simulink model "sampleModel7293_pp_1_1"  (R2018a)
settings: Solver=VariableStepAuto  StartTime=0.0  StopTime=10.0  RelTol=1e-3
undefined symbols (not defined in the file): DiscIntNeverNeededParam
libraries: simulink x367
(part 2 of 12)

== system sampleModel7293_pp_1_1/cfblk166 ==
  cfblk1 : Inport
  Action Port : ActionPort  ActionType=then
  cfblk10 : UnitDelay  SampleTime=-1
  cfblk3 : DiscreteTransferFcn
  cfblk4 : DiscreteFir
  cfblk5 : Subsystem  TreatAsAtomicUnit=on
  cfblk6 : UnitDelay  SampleTime=-1
  cfblk7 : Subsystem  TreatAsAtomicUnit=on
  cfblk8 : simulink/Discrete/Transfer Fcn Real Zero  ZeroZ=0.75  ICPrevInput=0.0  DoSatur=off
      settings: SourceProductName=Simulink  SourceProductBaseCode=SL
  cfblk9 : DiscreteFilter
  cyemi_{96..103} (8 alike) : DataTypeConversion  OutDataTypeStr=double
  emi_1695 : Subsystem  TreatAsAtomicUnit=on
  emi_1697 : If  IfExpression=Inf <= u1
  emi_1698 : DataTypeConversion  OutDataTypeStr=double
  emi_1838 : Subsystem  TreatAsAtomicUnit=on
  emi_1840 : If  IfExpression=Inf <= u1
  emi_1841 : DataTypeConversion  OutDataTypeStr=double
  cfblk2 : Outport
  cfblk11 : Outport  Port=2
  cfblk12 : Outport  Port=3
  wires:
  cfblk4/1 -> cfblk12/1
  cyemi_96/1 -> cfblk10/1
  cfblk8/1 -> cyemi_96/1
  cyemi_97/1 -> cfblk3/1
  cfblk10/1 -> cyemi_97/1, emi_1698/1
  cyemi_98/1 -> cfblk4/1
  cfblk3/1 -> cyemi_98/1, emi_1841/1
  cfblk1/1 -> cyemi_99/1
  cyemi_100/1 -> cfblk6/1
  cfblk9/1 -> cyemi_100/1
  cyemi_102/1 -> cfblk8/1
  cfblk6/1 -> cyemi_102/1
  cyemi_103/1 -> cfblk9/1
  cyemi_99/1 -> cfblk5/1(emi_1693)
  cfblk5/1(emi_1694) -> cyemi_103/1, cyemi_101/1, cfblk2/1
  emi_1697/1 -> cfblk5/Action
  emi_1697/2 -> emi_1695/Action
  emi_1698/1 -> emi_1697/1
  cyemi_101/1 -> cfblk7/1(emi_1836)
  cfblk7/1(emi_1837) -> cfblk11/1
  emi_1840/1 -> cfblk7/Action
  emi_1840/2 -> emi_1838/Action
  emi_1841/1 -> emi_1840/1

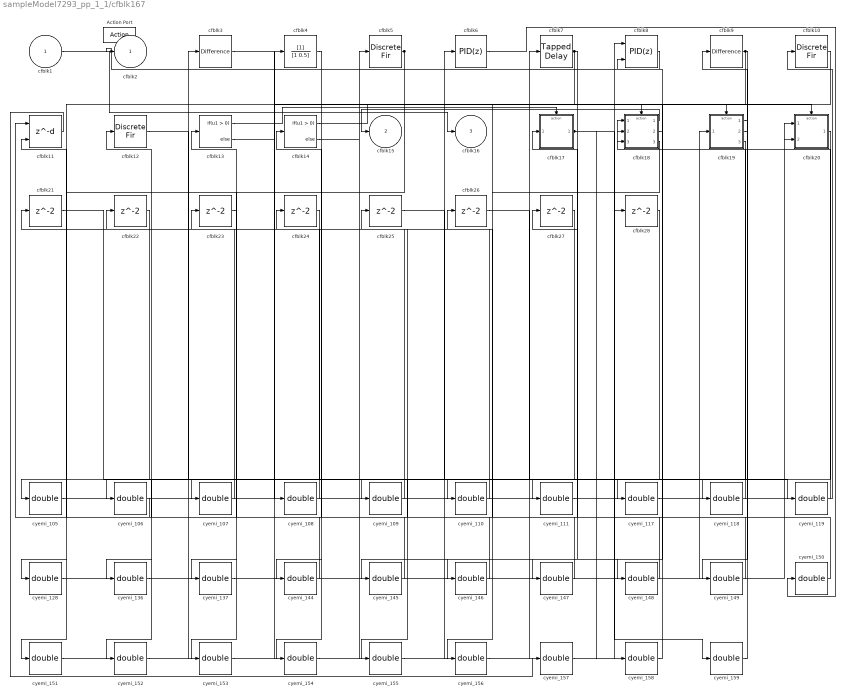
== system sampleModel7293_pp_1_1/cfblk167 ==
  cfblk1 : Inport
  Action Port : ActionPort  ActionType=else
  cfblk10 : DiscreteFir
  cfblk11 : Delay  DelayLengthSource=Input port
      settings: InputPortMap=u0,p1
  cfblk12 : DiscreteFir
  cfblk13 : If  SampleTime=1
  cfblk14 : If  SampleTime=1
  cfblk17 : Subsystem  TreatAsAtomicUnit=on
  cfblk18 : Subsystem  TreatAsAtomicUnit=on
  cfblk19 : Subsystem  TreatAsAtomicUnit=on
  cfblk20 : Subsystem  TreatAsAtomicUnit=on
  cfblk{21..28} (8 alike) : Delay
  cfblk3 : simulink/Discrete/Difference  ICPrevInput=0.0  OutMin=[]  OutMax=[]  OutDataTypeStr=double  OutputDataTypeScalingMode=double  OutDataType=fixdt(1, 16)  OutScaling=2^-10  DoSatur=off
  cfblk4 : DiscreteFilter
  cfblk5 : DiscreteFir
  cfblk6 : simulink/Continuous/PID Controller  Controller=PID  TimeDomain=Discrete-time  SampleTime=-1  IntegratorMethod=Forward Euler  FilterMethod=Forward Euler  Form=Parallel  UseFilter=on  ControllerParametersSource=internal  P=1  I=1  D=0  N=100  InitialConditionSource=internal  InitialConditionForIntegrator=0  InitialConditionForFilter=0  ExternalReset=none  LimitOutput=off  UpperSaturationLimit=inf  LowerSaturationLimit=-inf  LinearizeAsGain=off  AntiWindupMode=none  Kb=1  TrackingMode=off  Kt=1  PParamMin=[]  PParamMax=[]  IParamMin=[]  IParamMax=[]  DParamMin=[]  DParamMax=[]  NParamMin=[]  NParamMax=[]  KbParamMin=[]  KbParamMax=[]  KtParamMin=[]  KtParamMax=[]  POutMin=[]  POutMax=[]  IOutMin=[]  IOutMax=[]  DOutMin=[]  DOutMax=[]  NOutMin=[]  NOutMax=[]  KbOutMin=[]  KbOutMax=[]  KtOutMin=[]  KtOutMax=[]  IntegratorOutMin=[]  IntegratorOutMax=[]  FilterOutMin=[]  FilterOutMax=[]  SumOutMin=[]  SumOutMax=[]  SumI1OutMin=[]  SumI1OutMax=[]  SumI2OutMin=[]  SumI2OutMax=[]  SumI3OutMin=[]  SumI3OutMax=[]  SumDOutMin=[]  SumDOutMax=[]  SaturationOutMin=[]  SaturationOutMax=[]  IntegratorContinuousStateAttributes=''  IntegratorStateMustResolveToSignalObject=off  IntegratorRTWStateStorageClass=Auto  FilterContinuousStateAttributes=''  FilterStateMustResolveToSignalObject=off  FilterRTWStateStorageClass=Auto  DifferentiatorICPrevScaledInput=0  DifferentiatorOutMin=[]  DifferentiatorOutMax=[]  FilterDiffOutCoefMin=[]  FilterDiffOutCoefMax=[]  SumDenOutMin=[]  SumDenOutMax=[]  SumNumOutMin=[]  SumNumOutMax=[]  ReciprocalOutMin=[]  ReciprocalOutMax=[]  DivideOutMin=[]  DivideOutMax=[]  TunerSelectOption=Transfer Function Based (PID Tuner App)
  cfblk7 : simulink/Discrete/Tapped Delay  vinit=0.0  samptime=-1  NumDelays=1  DelayOrder=Oldest  includeCurrent=off
  cfblk8 : simulink/Continuous/PID Controller (2DOF)  Controller=PID  TimeDomain=Discrete-time  SampleTime=-1  IntegratorMethod=Forward Euler  FilterMethod=Forward Euler  Form=Parallel  UseFilter=on  ControllerParametersSource=internal  P=1  I=1  D=0  N=100  b=1  c=1  InitialConditionSource=internal  InitialConditionForIntegrator=0  InitialConditionForFilter=0  ExternalReset=none  LimitOutput=off  UpperSaturationLimit=inf  LowerSaturationLimit=-inf  LinearizeAsGain=off  AntiWindupMode=none  Kb=1  TrackingMode=off  Kt=1  PParamMin=[]  PParamMax=[]  IParamMin=[]  IParamMax=[]  DParamMin=[]  DParamMax=[]  NParamMin=[]  NParamMax=[]  bParamMin=[]  bParamMax=[]  cParamMin=[]  cParamMax=[]  KbParamMin=[]  KbParamMax=[]  KtParamMin=[]  KtParamMax=[]  POutMin=[]  POutMax=[]  IOutMin=[]  IOutMax=[]  DOutMin=[]  DOutMax=[]  NOutMin=[]  NOutMax=[]  bOutMin=[]  bOutMax=[]  cOutMin=[]  cOutMax=[]  KbOutMin=[]  KbOutMax=[]  KtOutMin=[]  KtOutMax=[]  IntegratorOutMin=[]  IntegratorOutMax=[]  FilterOutMin=[]  FilterOutMax=[]  SumOutMin=[]  SumOutMax=[]  Sum1OutMin=[]  Sum1OutMax=[]  Sum2OutMin=[]  Sum2OutMax=[]  Sum3OutMin=[]  Sum3OutMax=[]  SumI1OutMin=[]  SumI1OutMax=[]  SumI2OutMin=[]  SumI2OutMax=[]  SumI3OutMin=[]  SumI3OutMax=[]  SumDOutMin=[]  SumDOutMax=[]  SaturationOutMin=[]  SaturationOutMax=[]  IntegratorContinuousStateAttributes=''  IntegratorStateMustResolveToSignalObject=off  IntegratorRTWStateStorageClass=Auto  FilterContinuousStateAttributes=''  FilterStateMustResolveToSignalObject=off  FilterRTWStateStorageClass=Auto  DifferentiatorICPrevScaledInput=0  DifferentiatorOutMin=[]  DifferentiatorOutMax=[]  FilterDiffOutCoefMin=[]  FilterDiffOutCoefMax=[]  SumDenOutMin=[]  SumDenOutMax=[]  SumNumOutMin=[]  SumNumOutMax=[]  ReciprocalOutMin=[]  ReciprocalOutMax=[]  DivideOutMin=[]  DivideOutMax=[]  TunerSelectOption=Transfer Function Based (PID Tuner App)
  cfblk9 : simulink/Discrete/Difference  ICPrevInput=0.0  OutMin=[]  OutMax=[]  OutDataTypeStr=double  OutputDataTypeScalingMode=double  OutDataType=fixdt(1, 16)  OutScaling=2^-10  DoSatur=off
  cyemi_{105..111,117..119,128,136..137,144..159} (29 alike) : DataTypeConversion  OutDataTypeStr=double
  cfblk2 : Outport
  cfblk15 : Outport  Port=2
  cfblk16 : Outport  Port=3
  wires:
  cfblk1/1 -> cfblk16/1
  cfblk8/1 -> cfblk2/1
  cfblk17/1(cfblk2) -> cyemi_158/1, cyemi_159/1
  cfblk7/1 -> cyemi_111/1, cyemi_151/1
  cfblk18/1(cfblk2) -> cfblk15/1
  cfblk5/1 -> cyemi_105/1, cyemi_107/1
  cfblk9/1 -> cyemi_144/1, cyemi_148/1, cyemi_149/1
  cfblk13/1 -> cfblk17/Action
  cfblk13/2 -> cfblk18/Action
  cfblk14/1 -> cfblk19/Action
  cfblk14/2 -> cfblk20/Action
  cyemi_105/1 -> cfblk10/1
  cyemi_106/1 -> cfblk11/1
  cfblk19/1(cfblk2) -> cyemi_106/1
  cyemi_107/1 -> cfblk11/2
  cyemi_108/1 -> cfblk12/1
  cfblk3/1 -> cyemi_108/1
  cyemi_109/1 -> cfblk13/1
  cfblk19/2(cfblk8) -> cyemi_109/1
  cyemi_110/1 -> cfblk14/1
  cfblk12/1 -> cyemi_110/1
  cyemi_111/1 -> cfblk17/1(cfblk1)
  cyemi_117/1 -> cfblk18/1(cfblk1)
  cfblk21/1 -> cyemi_117/1
  cyemi_118/1 -> cfblk18/2(cfblk10)
  cfblk25/1 -> cyemi_118/1
  cyemi_119/1 -> cfblk18/3(cfblk11)
  cfblk26/1 -> cyemi_119/1
  cyemi_128/1 -> cfblk19/1(cfblk1)
  cfblk22/1 -> cyemi_128/1
  cyemi_136/1 -> cfblk20/1(cfblk1)
  cfblk27/1 -> cyemi_136/1
  cyemi_137/1 -> cfblk20/2(cfblk7)
  cfblk23/1 -> cyemi_137/1
  cyemi_144/1 -> cfblk21/1
  cyemi_145/1 -> cfblk22/1
  cfblk18/2(cfblk12) -> cyemi_145/1
  cyemi_146/1 -> cfblk23/1
  cfblk18/3(cfblk13) -> cyemi_146/1
  cyemi_147/1 -> cfblk24/1
  cfblk20/1(cfblk2) -> cyemi_147/1
  cyemi_148/1 -> cfblk25/1
  cyemi_149/1 -> cfblk26/1
  cyemi_150/1 -> cfblk27/1
  cfblk6/1 -> cyemi_150/1
  cyemi_151/1 -> cfblk28/1
  cyemi_152/1 -> cfblk3/1
  cfblk24/1 -> cyemi_152/1
  cyemi_153/1 -> cfblk4/1
  cfblk28/1 -> cyemi_153/1
  cyemi_154/1 -> cfblk5/1
  cfblk4/1 -> cyemi_154/1
  cyemi_155/1 -> cfblk6/1
  cfblk19/3(cfblk9) -> cyemi_155/1
  cyemi_156/1 -> cfblk7/1
  cfblk10/1 -> cyemi_156/1
  cyemi_157/1 -> cfblk8/1
  cfblk11/1 -> cyemi_157/1
  cyemi_158/1 -> cfblk8/2
  cyemi_159/1 -> cfblk9/1

== system sampleModel7293_pp_1_1/cfblk168 ==
  cfblk1 : Inport
  Action Port : ActionPort  ActionType=then
  cfblk3 : DiscreteStateSpace  SampleTime=-1
  cfblk4 : simulink/Continuous/PID Controller  Controller=PID  TimeDomain=Discrete-time  SampleTime=-1  IntegratorMethod=Forward Euler  FilterMethod=Forward Euler  Form=Parallel  UseFilter=on  ControllerParametersSource=internal  P=1  I=1  D=0  N=100  InitialConditionSource=internal  InitialConditionForIntegrator=0  InitialConditionForFilter=0  ExternalReset=none  LimitOutput=off  UpperSaturationLimit=inf  LowerSaturationLimit=-inf  LinearizeAsGain=off  AntiWindupMode=none  Kb=1  TrackingMode=off  Kt=1  PParamMin=[]  PParamMax=[]  IParamMin=[]  IParamMax=[]  DParamMin=[]  DParamMax=[]  NParamMin=[]  NParamMax=[]  KbParamMin=[]  KbParamMax=[]  KtParamMin=[]  KtParamMax=[]  POutMin=[]  POutMax=[]  IOutMin=[]  IOutMax=[]  DOutMin=[]  DOutMax=[]  NOutMin=[]  NOutMax=[]  KbOutMin=[]  KbOutMax=[]  KtOutMin=[]  KtOutMax=[]  IntegratorOutMin=[]  IntegratorOutMax=[]  FilterOutMin=[]  FilterOutMax=[]  SumOutMin=[]  SumOutMax=[]  SumI1OutMin=[]  SumI1OutMax=[]  SumI2OutMin=[]  SumI2OutMax=[]  SumI3OutMin=[]  SumI3OutMax=[]  SumDOutMin=[]  SumDOutMax=[]  SaturationOutMin=[]  SaturationOutMax=[]  IntegratorContinuousStateAttributes=''  IntegratorStateMustResolveToSignalObject=off  IntegratorRTWStateStorageClass=Auto  FilterContinuousStateAttributes=''  FilterStateMustResolveToSignalObject=off  FilterRTWStateStorageClass=Auto  DifferentiatorICPrevScaledInput=0  DifferentiatorOutMin=[]  DifferentiatorOutMax=[]  FilterDiffOutCoefMin=[]  FilterDiffOutCoefMax=[]  SumDenOutMin=[]  SumDenOutMax=[]  SumNumOutMin=[]  SumNumOutMax=[]  ReciprocalOutMin=[]  ReciprocalOutMax=[]  DivideOutMin=[]  DivideOutMax=[]  TunerSelectOption=Transfer Function Based (PID Tuner App)
  cfblk5 : DiscreteStateSpace  SampleTime=-1
  cfblk6 : DiscreteFir
  cfblk7 : Subsystem  TreatAsAtomicUnit=on
  cfblk9 : Delay
  cyemi_{161..167} (7 alike) : DataTypeConversion  OutDataTypeStr=double
  emi_1145 : Subsystem  TreatAsAtomicUnit=on
  emi_1147 : If  IfExpression=Inf <= u1
  emi_1148 : DataTypeConversion  OutDataTypeStr=double
  cfblk2 : Outport
  cfblk8 : Outport  Port=2
  wires:
  cfblk4/1 -> cfblk8/1
  cfblk6/1 -> cfblk2/1, cyemi_165/1, cyemi_166/1
  cyemi_161/1 -> cfblk3/1
  cfblk9/1 -> cyemi_161/1
  cyemi_162/1 -> cfblk4/1
  cfblk5/1 -> cyemi_162/1
  cyemi_163/1 -> cfblk5/1
  cfblk1/1 -> cyemi_163/1
  cyemi_164/1 -> cfblk6/1
  cfblk3/1 -> cyemi_164/1, emi_1148/1
  cyemi_167/1 -> cfblk9/1
  cyemi_165/1 -> cfblk7/1(emi_1142)
  cyemi_166/1 -> cfblk7/2(emi_1143)
  cfblk7/1(emi_1144) -> cyemi_167/1
  emi_1147/1 -> cfblk7/Action
  emi_1147/2 -> emi_1145/Action
  emi_1148/1 -> emi_1147/1

== system sampleModel7293_pp_1_1/cfblk169 ==
  cfblk1 : Inport
  cfblk12 : Inport  Port=2
  Action Port : ActionPort  ActionType=else
  cfblk10 : Delay
  cfblk11 : DiscreteFir
  cfblk3 : Subsystem  TreatAsAtomicUnit=on
  cfblk4 : simulink/Continuous/PID Controller  Controller=PID  TimeDomain=Discrete-time  SampleTime=-1  IntegratorMethod=Forward Euler  FilterMethod=Forward Euler  Form=Parallel  UseFilter=on  ControllerParametersSource=internal  P=1  I=1  D=0  N=100  InitialConditionSource=internal  InitialConditionForIntegrator=0  InitialConditionForFilter=0  ExternalReset=none  LimitOutput=off  UpperSaturationLimit=inf  LowerSaturationLimit=-inf  LinearizeAsGain=off  AntiWindupMode=none  Kb=1  TrackingMode=off  Kt=1  PParamMin=[]  PParamMax=[]  IParamMin=[]  IParamMax=[]  DParamMin=[]  DParamMax=[]  NParamMin=[]  NParamMax=[]  KbParamMin=[]  KbParamMax=[]  KtParamMin=[]  KtParamMax=[]  POutMin=[]  POutMax=[]  IOutMin=[]  IOutMax=[]  DOutMin=[]  DOutMax=[]  NOutMin=[]  NOutMax=[]  KbOutMin=[]  KbOutMax=[]  KtOutMin=[]  KtOutMax=[]  IntegratorOutMin=[]  IntegratorOutMax=[]  FilterOutMin=[]  FilterOutMax=[]  SumOutMin=[]  SumOutMax=[]  SumI1OutMin=[]  SumI1OutMax=[]  SumI2OutMin=[]  SumI2OutMax=[]  SumI3OutMin=[]  SumI3OutMax=[]  SumDOutMin=[]  SumDOutMax=[]  SaturationOutMin=[]  SaturationOutMax=[]  IntegratorContinuousStateAttributes=''  IntegratorStateMustResolveToSignalObject=off  IntegratorRTWStateStorageClass=Auto  FilterContinuousStateAttributes=''  FilterStateMustResolveToSignalObject=off  FilterRTWStateStorageClass=Auto  DifferentiatorICPrevScaledInput=0  DifferentiatorOutMin=[]  DifferentiatorOutMax=[]  FilterDiffOutCoefMin=[]  FilterDiffOutCoefMax=[]  SumDenOutMin=[]  SumDenOutMax=[]  SumNumOutMin=[]  SumNumOutMax=[]  ReciprocalOutMin=[]  ReciprocalOutMax=[]  DivideOutMin=[]  DivideOutMax=[]  TunerSelectOption=Transfer Function Based (PID Tuner App)
  cfblk5 : Subsystem  TreatAsAtomicUnit=on
  cfblk6 : Delay  DelayLengthSource=Input port
      settings: InputPortMap=u0,p1
  cfblk7 : Subsystem  TreatAsAtomicUnit=on
  cfblk8 : Subsystem  TreatAsAtomicUnit=on
  cfblk9 : Subsystem  TreatAsAtomicUnit=on
  cyemi_{170..180} (11 alike) : DataTypeConversion  OutDataTypeStr=double
  emi_1130 : Subsystem  TreatAsAtomicUnit=on
  emi_1132 : If  IfExpression=0 <= u1
  emi_{299,493,830,1133,1981} (5 alike) : DataTypeConversion  OutDataTypeStr=double
  emi_1978 : Subsystem  TreatAsAtomicUnit=on
  emi_1980 : If  IfExpression=0 <= u1
  emi_296 : Subsystem  TreatAsAtomicUnit=on
  emi_298 : If  IfExpression=-4.554546e-01 <= u1
  emi_490 : Subsystem  TreatAsAtomicUnit=on
  emi_492 : If  IfExpression=-4.554546e-01 <= u1
  emi_827 : Subsystem  TreatAsAtomicUnit=on
  emi_829 : If  IfExpression=0 <= u1
  cfblk2 : Outport
  cfblk13 : Outport  Port=2
  cfblk14 : Outport  Port=3
  wires:
  cfblk12/1 -> cyemi_171/1, cyemi_179/1, cyemi_180/1
  cfblk6/1 -> cfblk14/1, emi_1981/1
  cyemi_170/1 -> cfblk10/1
  cfblk1/1 -> cyemi_170/1
  cyemi_171/1 -> cfblk11/1
  cfblk4/1 -> cyemi_172/1
  cyemi_173/1 -> cfblk4/1
  cyemi_175/1 -> cfblk6/1
  cyemi_176/1 -> cfblk6/2
  cfblk10/1 -> cyemi_176/1
  cfblk11/1 -> cyemi_178/1, emi_299/1, emi_493/1
  cyemi_180/1 -> cfblk9/1(emi_294)
  cfblk9/1(emi_295) -> cyemi_177/1, cyemi_173/1
  emi_298/1 -> cfblk9/Action
  emi_298/2 -> emi_296/Action
  emi_299/1 -> emi_298/1
  cyemi_178/1 -> cfblk8/1(emi_487)
  cyemi_179/1 -> cfblk8/2(emi_488)
  cfblk8/1(emi_489) -> cyemi_174/1
  emi_492/1 -> cfblk8/Action
  emi_492/2 -> emi_490/Action
  emi_493/1 -> emi_492/1
  cyemi_174/1 -> cfblk5/1(emi_825)
  cfblk5/1(emi_826) -> cfblk2/1
  emi_829/1 -> cfblk5/Action
  emi_829/2 -> emi_827/Action
  emi_830/1 -> emi_829/1
  cyemi_172/1 -> cfblk3/1(emi_1128)
  cfblk3/1(emi_1129) -> cfblk13/1
  emi_1132/1 -> cfblk3/Action
  emi_1132/2 -> emi_1130/Action
  emi_1133/1 -> emi_1132/1
  cyemi_177/1 -> cfblk7/1(emi_1976)
  cfblk7/1(emi_1977) -> emi_1133/1, emi_830/1, cyemi_175/1
  emi_1980/1 -> cfblk7/Action
  emi_1980/2 -> emi_1978/Action
  emi_1981/1 -> emi_1980/1

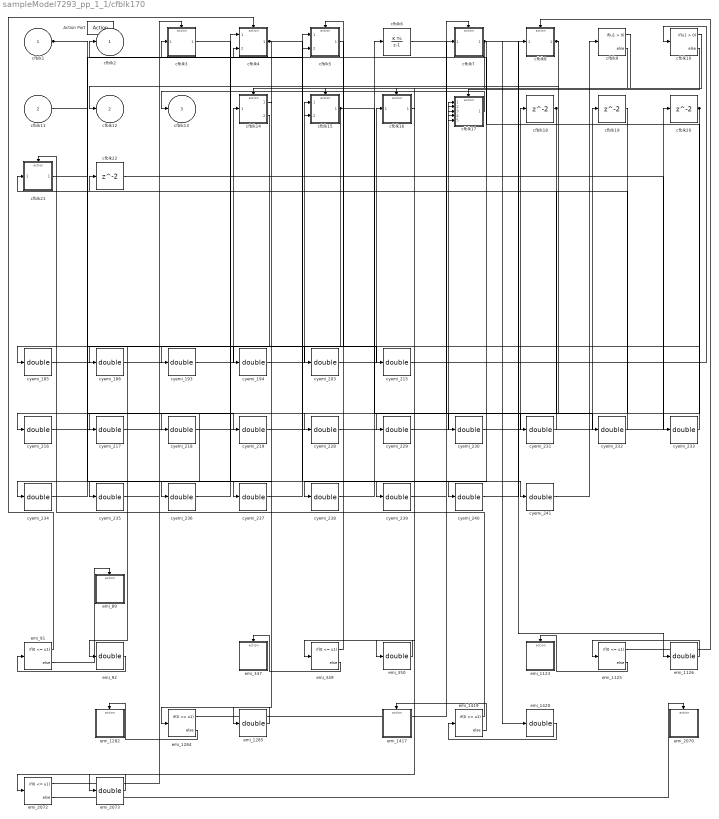
== system sampleModel7293_pp_1_1/cfblk170 ==
  cfblk1 : Inport
  cfblk11 : Inport  Port=2
  Action Port : ActionPort  ActionType=then
  cfblk10 : If  SampleTime=1
  cfblk14 : Subsystem  TreatAsAtomicUnit=on
  cfblk15 : Subsystem  TreatAsAtomicUnit=on
  cfblk16 : Subsystem  TreatAsAtomicUnit=on
  cfblk17 : Subsystem  TreatAsAtomicUnit=on
  cfblk{18..20,22} (4 alike) : Delay
  cfblk21 : Subsystem  TreatAsAtomicUnit=on
  cfblk3 : Subsystem  TreatAsAtomicUnit=on
  cfblk4 : Subsystem  TreatAsAtomicUnit=on
  cfblk5 : Subsystem  TreatAsAtomicUnit=on
  cfblk6 : DiscreteIntegrator  SampleTime=-1  OutDataTypeStr=double  ICPrevOutput=DiscIntNeverNeededParam  ICPrevScaledInput=DiscIntNeverNeededParam
  cfblk7 : Subsystem  TreatAsAtomicUnit=on
  cfblk8 : Subsystem  TreatAsAtomicUnit=on
  cfblk9 : If  SampleTime=1
  cyemi_{185..186,193..194,203,215..219,228..241} (24 alike) : DataTypeConversion  OutDataTypeStr=double
  emi_1123 : Subsystem  TreatAsAtomicUnit=on
  emi_{91,349,1125,1284,1419,2072} (6 alike) : If  IfExpression=0 <= u1
  emi_{92,350,1126,1285,1420,2073} (6 alike) : DataTypeConversion  OutDataTypeStr=double
  emi_1282 : Subsystem  TreatAsAtomicUnit=on
  emi_1417 : Subsystem  TreatAsAtomicUnit=on
  emi_2070 : Subsystem  TreatAsAtomicUnit=on
  emi_347 : Subsystem  TreatAsAtomicUnit=on
  emi_89 : Subsystem  TreatAsAtomicUnit=on
  cfblk2 : Outport
  cfblk12 : Outport  Port=2
  cfblk13 : Outport  Port=3
  wires:
  cfblk1/1 -> cyemi_219/1, cyemi_241/1
  cfblk17/1(cfblk2) -> cfblk13/1
  cfblk15/1(cfblk2) -> cyemi_230/1, cyemi_237/1
  cfblk9/1 -> cfblk14/Action
  cfblk9/2 -> cfblk15/Action
  cfblk10/1 -> cfblk16/Action
  cfblk10/2 -> cfblk17/Action
  cyemi_185/1 -> cfblk10/1
  cyemi_186/1 -> cfblk14/1(cfblk1)
  cfblk20/1 -> cyemi_186/1, emi_350/1, emi_1285/1
  cyemi_193/1 -> cfblk15/1(cfblk1)
  cfblk18/1 -> cyemi_193/1, emi_92/1
  cyemi_194/1 -> cfblk15/2(cfblk8)
  cyemi_203/1 -> cfblk16/1(cfblk1)
  cyemi_215/1 -> cfblk17/1(cfblk1)
  cfblk11/1 -> cyemi_215/1
  cyemi_216/1 -> cfblk17/2(cfblk10)
  cyemi_217/1 -> cfblk17/3(cfblk11)
  cyemi_218/1 -> cfblk17/4(cfblk12)
  cyemi_219/1 -> cfblk17/5(cfblk13)
  cyemi_228/1 -> cfblk18/1
  cyemi_229/1 -> cfblk19/1
  cfblk16/1(cfblk2) -> cyemi_229/1
  cyemi_230/1 -> cfblk20/1
  cyemi_232/1 -> cfblk22/1
  cfblk6/1 -> cyemi_232/1
  cfblk22/1 -> cyemi_233/1
  cfblk14/1(cfblk2) -> cyemi_234/1
  cfblk14/2(cfblk7) -> cyemi_235/1
  cfblk19/1 -> cyemi_236/1
  cyemi_238/1 -> cfblk6/1
  cyemi_241/1 -> cfblk9/1
  cyemi_234/1 -> cfblk4/1(emi_86)
  cyemi_235/1 -> cfblk4/2(emi_87)
  cfblk4/1(emi_88) -> cyemi_240/1, cyemi_216/1
  emi_91/1 -> cfblk4/Action
  emi_91/2 -> emi_89/Action
  emi_92/1 -> emi_91/1
  cyemi_236/1 -> cfblk5/1(emi_344)
  cyemi_237/1 -> cfblk5/2(emi_345)
  cfblk5/1(emi_346) -> cyemi_185/1
  emi_349/1 -> cfblk5/Action
  emi_349/2 -> emi_347/Action
  emi_350/1 -> emi_349/1
  cyemi_240/1 -> cfblk8/1(emi_1121)
  cfblk8/1(emi_1122) -> cyemi_231/1, cyemi_228/1, cyemi_218/1, cfblk12/1
  emi_1125/1 -> cfblk8/Action
  emi_1125/2 -> emi_1123/Action
  emi_1126/1 -> emi_1125/1
  cyemi_239/1 -> cfblk7/1(emi_1280)
  cfblk7/1(emi_1281) -> emi_1126/1, cyemi_238/1, cyemi_217/1, cyemi_203/1, cfblk2/1, emi_1420/1, emi_2073/1
  emi_1284/1 -> cfblk7/Action
  emi_1284/2 -> emi_1282/Action
  emi_1285/1 -> emi_1284/1
  cyemi_231/1 -> cfblk21/1(emi_1415)
  cfblk21/1(emi_1416) -> cyemi_194/1
  emi_1419/1 -> cfblk21/Action
  emi_1419/2 -> emi_1417/Action
  emi_1420/1 -> emi_1419/1
  cyemi_233/1 -> cfblk3/1(emi_2068)
  cfblk3/1(emi_2069) -> cyemi_239/1
  emi_2072/1 -> cfblk3/Action
  emi_2072/2 -> emi_2070/Action
  emi_2073/1 -> emi_2072/1

== system sampleModel7293_pp_1_1/cfblk171 ==
  cfblk1 : Inport
  Action Port : ActionPort  ActionType=else
  cfblk10 : Subsystem  TreatAsAtomicUnit=on
  cfblk11 : Subsystem  TreatAsAtomicUnit=on
  cfblk12 : Delay
  cfblk13 : Delay
  cfblk14 : Delay
  cfblk15 : Subsystem  TreatAsAtomicUnit=on
  cfblk3 : DiscreteFilter
  cfblk4 : Subsystem  TreatAsAtomicUnit=on
  cfblk5 : Subsystem  TreatAsAtomicUnit=on
  cfblk6 : DiscreteStateSpace  SampleTime=-1
  cfblk7 : simulink/Continuous/PID Controller  Controller=PID  TimeDomain=Discrete-time  SampleTime=-1  IntegratorMethod=Forward Euler  FilterMethod=Forward Euler  Form=Parallel  UseFilter=on  ControllerParametersSource=internal  P=1  I=1  D=0  N=100  InitialConditionSource=internal  InitialConditionForIntegrator=0  InitialConditionForFilter=0  ExternalReset=none  LimitOutput=off  UpperSaturationLimit=inf  LowerSaturationLimit=-inf  LinearizeAsGain=off  AntiWindupMode=none  Kb=1  TrackingMode=off  Kt=1  PParamMin=[]  PParamMax=[]  IParamMin=[]  IParamMax=[]  DParamMin=[]  DParamMax=[]  NParamMin=[]  NParamMax=[]  KbParamMin=[]  KbParamMax=[]  KtParamMin=[]  KtParamMax=[]  POutMin=[]  POutMax=[]  IOutMin=[]  IOutMax=[]  DOutMin=[]  DOutMax=[]  NOutMin=[]  NOutMax=[]  KbOutMin=[]  KbOutMax=[]  KtOutMin=[]  KtOutMax=[]  IntegratorOutMin=[]  IntegratorOutMax=[]  FilterOutMin=[]  FilterOutMax=[]  SumOutMin=[]  SumOutMax=[]  SumI1OutMin=[]  SumI1OutMax=[]  SumI2OutMin=[]  SumI2OutMax=[]  SumI3OutMin=[]  SumI3OutMax=[]  SumDOutMin=[]  SumDOutMax=[]  SaturationOutMin=[]  SaturationOutMax=[]  IntegratorContinuousStateAttributes=''  IntegratorStateMustResolveToSignalObject=off  IntegratorRTWStateStorageClass=Auto  FilterContinuousStateAttributes=''  FilterStateMustResolveToSignalObject=off  FilterRTWStateStorageClass=Auto  DifferentiatorICPrevScaledInput=0  DifferentiatorOutMin=[]  DifferentiatorOutMax=[]  FilterDiffOutCoefMin=[]  FilterDiffOutCoefMax=[]  SumDenOutMin=[]  SumDenOutMax=[]  SumNumOutMin=[]  SumNumOutMax=[]  ReciprocalOutMin=[]  ReciprocalOutMax=[]  DivideOutMin=[]  DivideOutMax=[]  TunerSelectOption=Transfer Function Based (PID Tuner App)
  cfblk8 : If  SampleTime=1
  cyemi_{243,262..264,268..277} (14 alike) : DataTypeConversion  OutDataTypeStr=double
  emi_173 : Subsystem  TreatAsAtomicUnit=on
  emi_175 : If  IfExpression=Inf <= u1
  emi_176 : DataTypeConversion  OutDataTypeStr=double
  emi_1943 : Subsystem  TreatAsAtomicUnit=on
  emi_1945 : If  IfExpression=Inf <= u1
  emi_1946 : DataTypeConversion  OutDataTypeStr=double
  emi_676 : Subsystem  TreatAsAtomicUnit=on
  emi_678 : If  IfExpression=Inf <= u1
  emi_679 : DataTypeConversion  OutDataTypeStr=double
  cfblk2 : Outport
  cfblk9 : Outport  Port=2
  wires:
  cfblk3/1 -> cyemi_269/1, cyemi_270/1
  cfblk11/2(cfblk8) -> cfblk9/1, cfblk2/1
  cfblk8/1 -> cfblk10/Action
  cfblk8/2 -> cfblk11/Action
  cyemi_243/1 -> cfblk10/1(cfblk1)
  cfblk12/1 -> cyemi_243/1
  cyemi_262/1 -> cfblk11/1(cfblk1)
  cfblk1/1 -> cyemi_262/1
  cyemi_263/1 -> cfblk11/2(cfblk6)
  cfblk13/1 -> cyemi_263/1, emi_176/1
  cyemi_264/1 -> cfblk11/3(cfblk7)
  cfblk14/1 -> cyemi_264/1
  cyemi_268/1 -> cfblk12/1
  cyemi_269/1 -> cfblk13/1
  cyemi_270/1 -> cfblk14/1
  cfblk10/2(cfblk16) -> cyemi_271/1
  cyemi_272/1 -> cfblk3/1
  cfblk10/1(cfblk2) -> cyemi_272/1
  cfblk6/1 -> cyemi_273/1, emi_679/1, emi_1946/1
  cfblk11/1(cfblk2) -> cyemi_274/1
  cyemi_275/1 -> cfblk6/1
  cfblk7/1 -> cyemi_275/1
  cyemi_276/1 -> cfblk7/1
  cyemi_277/1 -> cfblk8/1
  cyemi_274/1 -> cfblk5/1(emi_171)
  cfblk5/1(emi_172) -> cyemi_276/1
  emi_175/1 -> cfblk5/Action
  emi_175/2 -> emi_173/Action
  emi_176/1 -> emi_175/1
  cyemi_273/1 -> cfblk4/1(emi_674)
  cfblk4/1(emi_675) -> cyemi_268/1
  emi_678/1 -> cfblk4/Action
  emi_678/2 -> emi_676/Action
  emi_679/1 -> emi_678/1
  cyemi_271/1 -> cfblk15/1(emi_1941)
  cfblk15/1(emi_1942) -> cyemi_277/1
  emi_1945/1 -> cfblk15/Action
  emi_1945/2 -> emi_1943/Action
  emi_1946/1 -> emi_1945/1

== system sampleModel7293_pp_1_1/cfblk172 ==
  cfblk1 : Inport
  Action Port : ActionPort  ActionType=then
  cfblk12 : Delay
  cfblk3 : DiscreteFilter
  cfblk4 : simulink/Discrete/Transfer Fcn Lead or Lag  PoleZ=0.95  ZeroZ=0.75  ICPrevOutput=0.0  ICPrevInput=0.0  DoSatur=off
      settings: SourceProductName=Simulink  SourceProductBaseCode=SL
  cfblk5 : Delay  ShowEnablePort=on
      settings: InputPortMap=u0,e6
  cfblk6 : simulink/Discrete/Transfer Fcn First Order  PoleZ=0.95  ICPrevOutput=0.0  DoSatur=off
      settings: SourceProductName=Simulink
  cfblk7 : Subsystem  TreatAsAtomicUnit=on
  cfblk8 : DiscreteFir
  cfblk9 : simulink/Continuous/PID Controller  Controller=PID  TimeDomain=Discrete-time  SampleTime=-1  IntegratorMethod=Forward Euler  FilterMethod=Forward Euler  Form=Parallel  UseFilter=on  ControllerParametersSource=internal  P=1  I=1  D=0  N=100  InitialConditionSource=internal  InitialConditionForIntegrator=0  InitialConditionForFilter=0  ExternalReset=none  LimitOutput=off  UpperSaturationLimit=inf  LowerSaturationLimit=-inf  LinearizeAsGain=off  AntiWindupMode=none  Kb=1  TrackingMode=off  Kt=1  PParamMin=[]  PParamMax=[]  IParamMin=[]  IParamMax=[]  DParamMin=[]  DParamMax=[]  NParamMin=[]  NParamMax=[]  KbParamMin=[]  KbParamMax=[]  KtParamMin=[]  KtParamMax=[]  POutMin=[]  POutMax=[]  IOutMin=[]  IOutMax=[]  DOutMin=[]  DOutMax=[]  NOutMin=[]  NOutMax=[]  KbOutMin=[]  KbOutMax=[]  KtOutMin=[]  KtOutMax=[]  IntegratorOutMin=[]  IntegratorOutMax=[]  FilterOutMin=[]  FilterOutMax=[]  SumOutMin=[]  SumOutMax=[]  SumI1OutMin=[]  SumI1OutMax=[]  SumI2OutMin=[]  SumI2OutMax=[]  SumI3OutMin=[]  SumI3OutMax=[]  SumDOutMin=[]  SumDOutMax=[]  SaturationOutMin=[]  SaturationOutMax=[]  IntegratorContinuousStateAttributes=''  IntegratorStateMustResolveToSignalObject=off  IntegratorRTWStateStorageClass=Auto  FilterContinuousStateAttributes=''  FilterStateMustResolveToSignalObject=off  FilterRTWStateStorageClass=Auto  DifferentiatorICPrevScaledInput=0  DifferentiatorOutMin=[]  DifferentiatorOutMax=[]  FilterDiffOutCoefMin=[]  FilterDiffOutCoefMax=[]  SumDenOutMin=[]  SumDenOutMax=[]  SumNumOutMin=[]  SumNumOutMax=[]  ReciprocalOutMin=[]  ReciprocalOutMax=[]  DivideOutMin=[]  DivideOutMax=[]  TunerSelectOption=Transfer Function Based (PID Tuner App)
  cyemi_{279..287} (9 alike) : DataTypeConversion  OutDataTypeStr=double
  emi_975 : Subsystem  TreatAsAtomicUnit=on
  emi_977 : If  IfExpression=0 <= u1
  emi_978 : DataTypeConversion  OutDataTypeStr=double
  cfblk2 : Outport
  cfblk10 : Outport  Port=2
  cfblk11 : Outport  Port=3
  wires:
  cfblk3/1 -> cfblk2/1, cyemi_282/1
  cfblk9/1 -> cyemi_279/1, cyemi_286/1
  cfblk8/1 -> cfblk10/1, cyemi_281/1
  cyemi_279/1 -> cfblk12/1
  cyemi_280/1 -> cfblk3/1
  cfblk1/1 -> cyemi_280/1
  cyemi_281/1 -> cfblk4/1
  cyemi_282/1 -> cfblk5/1
  cyemi_283/1 -> cfblk5/2
  cfblk4/1 -> cyemi_283/1
  cyemi_284/1 -> cfblk6/1
  cfblk12/1 -> cyemi_284/1
  cfblk5/1 -> cyemi_285/1, emi_978/1
  cyemi_286/1 -> cfblk8/1
  cyemi_287/1 -> cfblk9/1
  cfblk6/1 -> cyemi_287/1
  cyemi_285/1 -> cfblk7/1(emi_973)
  cfblk7/1(emi_974) -> cfblk11/1
  emi_977/1 -> cfblk7/Action
  emi_977/2 -> emi_975/Action
  emi_978/1 -> emi_977/1

== system sampleModel7293_pp_1_1/cfblk173 ==
  cfblk1 : Inport
  Action Port : ActionPort  ActionType=else
  cfblk10 : DiscreteTransferFcn
  cfblk11 : If  SampleTime=1
  cfblk13 : Subsystem  TreatAsAtomicUnit=on
  cfblk14 : Subsystem  TreatAsAtomicUnit=on
  cfblk15 : Delay
  cfblk16 : Delay
  cfblk3 : DiscreteIntegrator  SampleTime=-1  OutDataTypeStr=double  ICPrevOutput=DiscIntNeverNeededParam  ICPrevScaledInput=DiscIntNeverNeededParam
  cfblk4 : DiscreteStateSpace  SampleTime=-1
  cfblk5 : Delay
  cfblk6 : DiscreteZeroPole  Poles=[0 0.5]  Gain=1  SampleTime=-1
  cfblk7 : simulink/Discrete/Difference  ICPrevInput=0.0  OutMin=[]  OutMax=[]  OutDataTypeStr=double  OutputDataTypeScalingMode=double  OutDataType=fixdt(1, 16)  OutScaling=2^-10  DoSatur=off
  cfblk8 : simulink/Discrete/Difference  ICPrevInput=0.0  OutMin=[]  OutMax=[]  OutDataTypeStr=double  OutputDataTypeScalingMode=double  OutDataType=fixdt(1, 16)  OutScaling=2^-10  DoSatur=off
  cfblk9 : DiscreteZeroPole  Poles=[0 0.5]  Gain=1  SampleTime=-1
  cyemi_{289..292,303..305,312..320} (16 alike) : DataTypeConversion  OutDataTypeStr=double
  cfblk2 : Outport
  cfblk12 : Outport  Port=2
  wires:
  cfblk1/1 -> cyemi_291/1, cyemi_317/1
  cfblk13/1(cfblk2) -> cfblk12/1
  cfblk8/1 -> cyemi_304/1, cyemi_315/1
  cfblk5/1 -> cyemi_289/1, cyemi_292/1, cyemi_305/1, cyemi_320/1
  cfblk7/1 -> cfblk2/1
  cfblk11/1 -> cfblk13/Action
  cfblk11/2 -> cfblk14/Action
  cyemi_289/1 -> cfblk10/1
  cyemi_290/1 -> cfblk11/1
  cfblk15/1 -> cyemi_290/1
  cyemi_291/1 -> cfblk13/1(cfblk1)
  cyemi_292/1 -> cfblk13/2(cfblk12)
  cyemi_303/1 -> cfblk14/1(cfblk1)
  cfblk4/1 -> cyemi_303/1
  cyemi_304/1 -> cfblk14/2(cfblk7)
  cyemi_305/1 -> cfblk14/3(cfblk8)
  cyemi_312/1 -> cfblk15/1
  cfblk14/1(cfblk2) -> cyemi_312/1
  cyemi_313/1 -> cfblk16/1
  cfblk10/1 -> cyemi_313/1
  cyemi_314/1 -> cfblk3/1
  cfblk6/1 -> cyemi_314/1
  cyemi_315/1 -> cfblk4/1
  cyemi_316/1 -> cfblk5/1
  cfblk16/1 -> cyemi_316/1
  cyemi_317/1 -> cfblk6/1
  cyemi_318/1 -> cfblk7/1
  cfblk9/1 -> cyemi_318/1
  cyemi_319/1 -> cfblk8/1
  cfblk3/1 -> cyemi_319/1
  cyemi_320/1 -> cfblk9/1

== system sampleModel7293_pp_1_1/cfblk174 ==
  cfblk1 : Inport
  Action Port : ActionPort  ActionType=then
  cfblk3 : Subsystem  TreatAsAtomicUnit=on
  cfblk4 : Delay  ShowEnablePort=on
      settings: InputPortMap=u0,e6
  cfblk5 : DiscreteZeroPole  Poles=[0 0.5]  Gain=1  SampleTime=-1
  cfblk6 : Subsystem  TreatAsAtomicUnit=on
  cfblk7 : DiscreteStateSpace  SampleTime=-1
  cfblk8 : simulink/Discrete/Transfer Fcn First Order  PoleZ=0.95  ICPrevOutput=0.0  DoSatur=off
      settings: SourceProductName=Simulink
  cyemi_{322..328} (7 alike) : DataTypeConversion  OutDataTypeStr=double
  emi_598 : Subsystem  TreatAsAtomicUnit=on
  emi_600 : If  IfExpression=Inf <= u1
  emi_601 : DataTypeConversion  OutDataTypeStr=double
  emi_619 : Subsystem  TreatAsAtomicUnit=on
  emi_621 : If  IfExpression=Inf <= u1
  emi_622 : DataTypeConversion  OutDataTypeStr=double
  cfblk2 : Outport
  cfblk9 : Outport  Port=2
  wires:
  cfblk7/1 -> cfblk9/1, emi_601/1
  cfblk1/1 -> cyemi_322/1, cyemi_328/1
  cfblk4/1 -> cfblk2/1, cyemi_325/1
  cyemi_323/1 -> cfblk4/1
  cyemi_324/1 -> cfblk4/2
  cyemi_325/1 -> cfblk5/1
  cfblk8/1 -> cyemi_326/1
  cyemi_327/1 -> cfblk7/1
  cfblk5/1 -> cyemi_327/1
  cyemi_328/1 -> cfblk8/1
  cyemi_326/1 -> cfblk6/1(emi_596)
  cfblk6/1(emi_597) -> cyemi_324/1, emi_622/1
  emi_600/1 -> cfblk6/Action
  emi_600/2 -> emi_598/Action
  emi_601/1 -> emi_600/1
  cyemi_322/1 -> cfblk3/1(emi_617)
  cfblk3/1(emi_618) -> cyemi_323/1
  emi_621/1 -> cfblk3/Action
  emi_621/2 -> emi_619/Action
  emi_622/1 -> emi_621/1

== system sampleModel7293_pp_1_1/cfblk175 ==
  cfblk1 : Inport
  cfblk11 : Inport  Port=2
  Action Port : ActionPort  ActionType=else
  cfblk10 : If  SampleTime=1
  cfblk16 : Subsystem  TreatAsAtomicUnit=on
  cfblk17 : Subsystem  TreatAsAtomicUnit=on
  cfblk18 : Delay
  cfblk19 : Delay
  cfblk3 : simulink/Continuous/PID Controller  Controller=PID  TimeDomain=Discrete-time  SampleTime=-1  IntegratorMethod=Forward Euler  FilterMethod=Forward Euler  Form=Parallel  UseFilter=on  ControllerParametersSource=internal  P=1  I=1  D=0  N=100  InitialConditionSource=internal  InitialConditionForIntegrator=0  InitialConditionForFilter=0  ExternalReset=none  LimitOutput=off  UpperSaturationLimit=inf  LowerSaturationLimit=-inf  LinearizeAsGain=off  AntiWindupMode=none  Kb=1  TrackingMode=off  Kt=1  PParamMin=[]  PParamMax=[]  IParamMin=[]  IParamMax=[]  DParamMin=[]  DParamMax=[]  NParamMin=[]  NParamMax=[]  KbParamMin=[]  KbParamMax=[]  KtParamMin=[]  KtParamMax=[]  POutMin=[]  POutMax=[]  IOutMin=[]  IOutMax=[]  DOutMin=[]  DOutMax=[]  NOutMin=[]  NOutMax=[]  KbOutMin=[]  KbOutMax=[]  KtOutMin=[]  KtOutMax=[]  IntegratorOutMin=[]  IntegratorOutMax=[]  FilterOutMin=[]  FilterOutMax=[]  SumOutMin=[]  SumOutMax=[]  SumI1OutMin=[]  SumI1OutMax=[]  SumI2OutMin=[]  SumI2OutMax=[]  SumI3OutMin=[]  SumI3OutMax=[]  SumDOutMin=[]  SumDOutMax=[]  SaturationOutMin=[]  SaturationOutMax=[]  IntegratorContinuousStateAttributes=''  IntegratorStateMustResolveToSignalObject=off  IntegratorRTWStateStorageClass=Auto  FilterContinuousStateAttributes=''  FilterStateMustResolveToSignalObject=off  FilterRTWStateStorageClass=Auto  DifferentiatorICPrevScaledInput=0  DifferentiatorOutMin=[]  DifferentiatorOutMax=[]  FilterDiffOutCoefMin=[]  FilterDiffOutCoefMax=[]  SumDenOutMin=[]  SumDenOutMax=[]  SumNumOutMin=[]  SumNumOutMax=[]  ReciprocalOutMin=[]  ReciprocalOutMax=[]  DivideOutMin=[]  DivideOutMax=[]  TunerSelectOption=Transfer Function Based (PID Tuner App)
  cfblk4 : simulink/Discrete/Tapped Delay  vinit=0.0  samptime=-1  NumDelays=1  DelayOrder=Oldest  includeCurrent=off
  cfblk5 : Subsystem  TreatAsAtomicUnit=on
  cfblk6 : Subsystem  TreatAsAtomicUnit=on
  cfblk7 : Subsystem  TreatAsAtomicUnit=on
  cfblk8 : Subsystem  TreatAsAtomicUnit=on
  cfblk9 : simulink/Continuous/PID Controller (2DOF)  Controller=PID  TimeDomain=Discrete-time  SampleTime=-1  IntegratorMethod=Forward Euler  FilterMethod=Forward Euler  Form=Parallel  UseFilter=on  ControllerParametersSource=internal  P=1  I=1  D=0  N=100  b=1  c=1  InitialConditionSource=internal  InitialConditionForIntegrator=0  InitialConditionForFilter=0  ExternalReset=none  LimitOutput=off  UpperSaturationLimit=inf  LowerSaturationLimit=-inf  LinearizeAsGain=off  AntiWindupMode=none  Kb=1  TrackingMode=off  Kt=1  PParamMin=[]  PParamMax=[]  IParamMin=[]  IParamMax=[]  DParamMin=[]  DParamMax=[]  NParamMin=[]  NParamMax=[]  bParamMin=[]  bParamMax=[]  cParamMin=[]  cParamMax=[]  KbParamMin=[]  KbParamMax=[]  KtParamMin=[]  KtParamMax=[]  POutMin=[]  POutMax=[]  IOutMin=[]  IOutMax=[]  DOutMin=[]  DOutMax=[]  NOutMin=[]  NOutMax=[]  bOutMin=[]  bOutMax=[]  cOutMin=[]  cOutMax=[]  KbOutMin=[]  KbOutMax=[]  KtOutMin=[]  KtOutMax=[]  IntegratorOutMin=[]  IntegratorOutMax=[]  FilterOutMin=[]  FilterOutMax=[]  SumOutMin=[]  SumOutMax=[]  Sum1OutMin=[]  Sum1OutMax=[]  Sum2OutMin=[]  Sum2OutMax=[]  Sum3OutMin=[]  Sum3OutMax=[]  SumI1OutMin=[]  SumI1OutMax=[]  SumI2OutMin=[]  SumI2OutMax=[]  SumI3OutMin=[]  SumI3OutMax=[]  SumDOutMin=[]  SumDOutMax=[]  SaturationOutMin=[]  SaturationOutMax=[]  IntegratorContinuousStateAttributes=''  IntegratorStateMustResolveToSignalObject=off  IntegratorRTWStateStorageClass=Auto  FilterContinuousStateAttributes=''  FilterStateMustResolveToSignalObject=off  FilterRTWStateStorageClass=Auto  DifferentiatorICPrevScaledInput=0  DifferentiatorOutMin=[]  DifferentiatorOutMax=[]  FilterDiffOutCoefMin=[]  FilterDiffOutCoefMax=[]  SumDenOutMin=[]  SumDenOutMax=[]  SumNumOutMin=[]  SumNumOutMax=[]  ReciprocalOutMin=[]  ReciprocalOutMax=[]  DivideOutMin=[]  DivideOutMax=[]  TunerSelectOption=Transfer Function Based (PID Tuner App)
  cyemi_{331..332,342..343,358..368} (15 alike) : DataTypeConversion  OutDataTypeStr=double
  emi_196 : Subsystem  TreatAsAtomicUnit=on
  emi_{198,319,506,991} (4 alike) : If  IfExpression=0 <= u1
  emi_{199,320,507,992} (4 alike) : DataTypeConversion  OutDataTypeStr=double
  emi_317 : Subsystem  TreatAsAtomicUnit=on
  emi_504 : Subsystem  TreatAsAtomicUnit=on
  emi_989 : Subsystem  TreatAsAtomicUnit=on
  cfblk2 : Outport
  cfblk12 : Outport  Port=2
  cfblk13 : Outport  Port=3
  cfblk14 : Outport  Port=4
  cfblk15 : Outport  Port=5
  wires:
  cfblk3/1 -> cfblk12/1, cyemi_332/1, cyemi_361/1
  cfblk9/1 -> cfblk2/1, cyemi_365/1
  cfblk17/1(cfblk2) -> cfblk15/1
  cfblk16/1(cfblk2) -> cfblk14/1
  cfblk11/1 -> cyemi_343/1, cyemi_363/1
  cfblk10/1 -> cfblk16/Action
  cfblk10/2 -> cfblk17/Action
  cyemi_331/1 -> cfblk10/1
  cfblk18/1 -> cyemi_331/1
  cyemi_332/1 -> cfblk16/1(cfblk1)
  cyemi_342/1 -> cfblk17/1(cfblk1)
  cyemi_343/1 -> cfblk17/2(cfblk14)
  cyemi_358/1 -> cfblk18/1
  cfblk17/2(cfblk15) -> cyemi_358/1
  cyemi_359/1 -> cfblk19/1
  cyemi_360/1 -> cfblk3/1
  cyemi_361/1 -> cfblk4/1
  cfblk4/1 -> cyemi_364/1, emi_199/1, emi_507/1
  cfblk1/1 -> cyemi_366/1
  cyemi_367/1 -> cfblk9/1
  cfblk19/1 -> cyemi_367/1, emi_992/1
  cyemi_368/1 -> cfblk9/2
  cyemi_362/1 -> cfblk5/1(emi_193)
  cyemi_363/1 -> cfblk5/2(emi_194)
  cfblk5/1(emi_195) -> cyemi_359/1
  emi_198/1 -> cfblk5/Action
  emi_198/2 -> emi_196/Action
  emi_199/1 -> emi_198/1
  cyemi_366/1 -> cfblk8/1(emi_315)
  cfblk8/1(emi_316) -> cyemi_360/1
  emi_319/1 -> cfblk8/Action
  emi_319/2 -> emi_317/Action
  emi_320/1 -> emi_319/1
  cyemi_364/1 -> cfblk6/1(emi_502)
  cfblk6/1(emi_503) -> cyemi_368/1
  emi_506/1 -> cfblk6/Action
  emi_506/2 -> emi_504/Action
  emi_507/1 -> emi_506/1
  cyemi_365/1 -> cfblk7/1(emi_987)
  cfblk7/1(emi_988) -> emi_320/1, cyemi_362/1, cyemi_342/1, cfblk13/1
  emi_991/1 -> cfblk7/Action
  emi_991/2 -> emi_989/Action
  emi_992/1 -> emi_991/1

== system sampleModel7293_pp_1_1/cfblk176 ==
  cfblk1 : Inport
  cfblk8 : Inport  Port=2
  cfblk9 : Inport  Port=3
  cfblk10 : Inport  Port=4
  cfblk11 : Inport  Port=5
  Action Port : ActionPort  ActionType=then
  cfblk3 : Delay  DelayLengthSource=Input port
      settings: InputPortMap=u0,p1
  cfblk4 : DiscreteZeroPole  Poles=[0 0.5]  Gain=1  SampleTime=-1
  cfblk5 : DiscreteTransferFcn
  cfblk6 : Delay  ShowEnablePort=on
      settings: InputPortMap=u0,e6
  cfblk7 : UnitDelay  SampleTime=-1
  cyemi_{374..380} (7 alike) : DataTypeConversion  OutDataTypeStr=double
  cfblk2 : Outport
  cfblk12 : Outport  Port=2
  wires:
  cfblk8/1 -> cfblk2/1
  cfblk6/1 -> cfblk12/1
  cyemi_374/1 -> cfblk3/1
  cfblk10/1 -> cyemi_374/1
  cyemi_375/1 -> cfblk3/2
  cfblk11/1 -> cyemi_375/1
  cyemi_376/1 -> cfblk4/1
  cfblk1/1 -> cyemi_376/1
  cyemi_377/1 -> cfblk5/1
  cfblk9/1 -> cyemi_377/1
  cyemi_378/1 -> cfblk6/1
  cfblk7/1 -> cyemi_378/1
  cyemi_379/1 -> cfblk6/2
  cfblk5/1 -> cyemi_379/1
  cyemi_380/1 -> cfblk7/1
  cfblk3/1 -> cyemi_380/1

== system sampleModel7293_pp_1_1/cfblk177 ==
  cfblk1 : Inport
  cfblk9 : Inport  Port=2
  cfblk10 : Inport  Port=3
  cfblk11 : Inport  Port=4
  Action Port : ActionPort  ActionType=else
  cfblk3 : Delay  ShowEnablePort=on
      settings: InputPortMap=u0,e6
  cfblk4 : simulink/Continuous/PID Controller (2DOF)  Controller=PID  TimeDomain=Discrete-time  SampleTime=-1  IntegratorMethod=Forward Euler  FilterMethod=Forward Euler  Form=Parallel  UseFilter=on  ControllerParametersSource=internal  P=1  I=1  D=0  N=100  b=1  c=1  InitialConditionSource=internal  InitialConditionForIntegrator=0  InitialConditionForFilter=0  ExternalReset=none  LimitOutput=off  UpperSaturationLimit=inf  LowerSaturationLimit=-inf  LinearizeAsGain=off  AntiWindupMode=none  Kb=1  TrackingMode=off  Kt=1  PParamMin=[]  PParamMax=[]  IParamMin=[]  IParamMax=[]  DParamMin=[]  DParamMax=[]  NParamMin=[]  NParamMax=[]  bParamMin=[]  bParamMax=[]  cParamMin=[]  cParamMax=[]  KbParamMin=[]  KbParamMax=[]  KtParamMin=[]  KtParamMax=[]  POutMin=[]  POutMax=[]  IOutMin=[]  IOutMax=[]  DOutMin=[]  DOutMax=[]  NOutMin=[]  NOutMax=[]  bOutMin=[]  bOutMax=[]  cOutMin=[]  cOutMax=[]  KbOutMin=[]  KbOutMax=[]  KtOutMin=[]  KtOutMax=[]  IntegratorOutMin=[]  IntegratorOutMax=[]  FilterOutMin=[]  FilterOutMax=[]  SumOutMin=[]  SumOutMax=[]  Sum1OutMin=[]  Sum1OutMax=[]  Sum2OutMin=[]  Sum2OutMax=[]  Sum3OutMin=[]  Sum3OutMax=[]  SumI1OutMin=[]  SumI1OutMax=[]  SumI2OutMin=[]  SumI2OutMax=[]  SumI3OutMin=[]  SumI3OutMax=[]  SumDOutMin=[]  SumDOutMax=[]  SaturationOutMin=[]  SaturationOutMax=[]  IntegratorContinuousStateAttributes=''  IntegratorStateMustResolveToSignalObject=off  IntegratorRTWStateStorageClass=Auto  FilterContinuousStateAttributes=''  FilterStateMustResolveToSignalObject=off  FilterRTWStateStorageClass=Auto  DifferentiatorICPrevScaledInput=0  DifferentiatorOutMin=[]  DifferentiatorOutMax=[]  FilterDiffOutCoefMin=[]  FilterDiffOutCoefMax=[]  SumDenOutMin=[]  SumDenOutMax=[]  SumNumOutMin=[]  SumNumOutMax=[]  ReciprocalOutMin=[]  ReciprocalOutMax=[]  DivideOutMin=[]  DivideOutMax=[]  TunerSelectOption=Transfer Function Based (PID Tuner App)
  cfblk5 : DiscreteFir
  cfblk6 : DiscreteFir
  cfblk7 : simulink/Discrete/Transfer Fcn Lead or Lag  PoleZ=0.95  ZeroZ=0.75  ICPrevOutput=0.0  ICPrevInput=0.0  DoSatur=off
      settings: SourceProductName=Simulink  SourceProductBaseCode=SL
  cfblk8 : Subsystem  TreatAsAtomicUnit=on
  cyemi_{385..392} (8 alike) : DataTypeConversion  OutDataTypeStr=double
  emi_52 : Subsystem  TreatAsAtomicUnit=on
  emi_54 : If  IfExpression=0 <= u1
  emi_55 : DataTypeConversion  OutDataTypeStr=double
  cfblk2 : Outport
  cfblk12 : Outport  Port=2
  cfblk13 : Outport  Port=3
  cfblk14 : Outport  Port=4
  wires:
  cfblk3/1 -> cfblk2/1
  cfblk9/1 -> cyemi_387/1, cyemi_392/1
  cfblk5/1 -> cfblk12/1, cfblk13/1
  cyemi_385/1 -> cfblk3/1
  cfblk4/1 -> cyemi_385/1
  cyemi_386/1 -> cfblk3/2
  cfblk7/1 -> cyemi_386/1
  cyemi_387/1 -> cfblk4/1
  cyemi_388/1 -> cfblk4/2
  cfblk10/1 -> cyemi_388/1
  cyemi_389/1 -> cfblk5/1
  cfblk11/1 -> cyemi_389/1
  cyemi_390/1 -> cfblk6/1
  cfblk1/1 -> cyemi_390/1
  cyemi_391/1 -> cfblk7/1
  cfblk6/1 -> cyemi_391/1, emi_55/1
  cyemi_392/1 -> cfblk8/1(emi_50)
  cfblk8/1(emi_51) -> cfblk14/1
  emi_54/1 -> cfblk8/Action
  emi_54/2 -> emi_52/Action
  emi_55/1 -> emi_54/1

== system sampleModel7293_pp_1_1/cfblk178 ==
  cfblk1 : Inport
  cfblk11 : Inport  Port=2
  Action Port : ActionPort  ActionType=then
  cfblk10 : simulink/Discrete/Transfer Fcn Real Zero  ZeroZ=0.75  ICPrevInput=0.0  DoSatur=off
      settings: SourceProductName=Simulink  SourceProductBaseCode=SL
  cfblk14 : Delay
  cfblk3 : Subsystem  TreatAsAtomicUnit=on
  cfblk4 : Subsystem  TreatAsAtomicUnit=on
  cfblk5 : simulink/Discrete/Transfer Fcn First Order  PoleZ=0.95  ICPrevOutput=0.0  DoSatur=off
      settings: SourceProductName=Simulink
  cfblk6 : UnitDelay  SampleTime=-1
  cfblk7 : DiscreteTransferFcn
  cfblk8 : DiscreteFir
  cfblk9 : Subsystem  TreatAsAtomicUnit=on
  cyemi_{395..403} (9 alike) : DataTypeConversion  OutDataTypeStr=double
  emi_1652 : Subsystem  TreatAsAtomicUnit=on
  emi_1654 : If  IfExpression=0 <= u1
  emi_1655 : DataTypeConversion  OutDataTypeStr=double
  emi_2021 : Subsystem  TreatAsAtomicUnit=on
  emi_2023 : If  IfExpression=0 <= u1
  emi_2024 : DataTypeConversion  OutDataTypeStr=double
  emi_748 : Subsystem  TreatAsAtomicUnit=on
  emi_750 : If  IfExpression=0 <= u1
  emi_751 : DataTypeConversion  OutDataTypeStr=double
  cfblk2 : Outport
  cfblk12 : Outport  Port=2
  cfblk13 : Outport  Port=3
  wires:
  cfblk1/1 -> cfblk13/1, cyemi_397/1
  cfblk10/1 -> cfblk12/1
  cyemi_395/1 -> cfblk10/1
  cfblk8/1 -> cyemi_395/1
  cyemi_396/1 -> cfblk14/1
  cfblk14/1 -> cyemi_398/1, emi_1655/1
  cyemi_399/1 -> cfblk5/1
  cyemi_400/1 -> cfblk6/1
  cfblk5/1 -> cyemi_400/1
  cyemi_401/1 -> cfblk7/1
  cfblk6/1 -> cyemi_401/1, emi_2024/1
  cyemi_402/1 -> cfblk8/1
  cfblk11/1 -> cyemi_402/1
  cfblk7/1 -> cyemi_403/1
  cyemi_398/1 -> cfblk4/1(emi_746)
  cfblk4/1(emi_747) -> cyemi_399/1
  emi_750/1 -> cfblk4/Action
  emi_750/2 -> emi_748/Action
  emi_751/1 -> emi_750/1
  cyemi_397/1 -> cfblk3/1(emi_1650)
  cfblk3/1(emi_1651) -> cfblk2/1
  emi_1654/1 -> cfblk3/Action
  emi_1654/2 -> emi_1652/Action
  emi_1655/1 -> emi_1654/1
  cyemi_403/1 -> cfblk9/1(emi_2019)
  cfblk9/1(emi_2020) -> emi_751/1, cyemi_396/1
  emi_2023/1 -> cfblk9/Action
  emi_2023/2 -> emi_2021/Action
  emi_2024/1 -> emi_2023/1

== system sampleModel7293_pp_1_1/cfblk179 ==
  cfblk1 : Inport
  cfblk11 : Inport  Port=2
  cfblk12 : Inport  Port=3
  Action Port : ActionPort  ActionType=else
  cfblk10 : DiscreteTransferFcn
  cfblk16 : Subsystem  TreatAsAtomicUnit=on
  cfblk17 : Delay
  cfblk3 : Delay
  cfblk4 : UnitDelay  SampleTime=-1
  cfblk5 : simulink/Discrete/Tapped Delay  vinit=0.0  samptime=-1  NumDelays=1  DelayOrder=Oldest  includeCurrent=off
  cfblk6 : Delay  ShowEnablePort=on
      settings: InputPortMap=u0,e6
  cfblk7 : Subsystem  TreatAsAtomicUnit=on
  cfblk8 : Subsystem  TreatAsAtomicUnit=on
  cfblk9 : Delay  ShowEnablePort=on
      settings: InputPortMap=u0,e6
  cyemi_{407..418} (12 alike) : DataTypeConversion  OutDataTypeStr=double
  emi_1289 : Subsystem  TreatAsAtomicUnit=on
  emi_1291 : If  IfExpression=0 <= u1
  emi_1292 : DataTypeConversion  OutDataTypeStr=double
  emi_1602 : Subsystem  TreatAsAtomicUnit=on
  emi_1604 : If  IfExpression=0 <= u1
  emi_1605 : DataTypeConversion  OutDataTypeStr=double
  emi_59 : Subsystem  TreatAsAtomicUnit=on
  emi_61 : If  IfExpression=0 <= u1
  emi_62 : DataTypeConversion  OutDataTypeStr=double
  cfblk2 : Outport
  cfblk13 : Outport  Port=2
  cfblk14 : Outport  Port=3
  cfblk15 : Outport  Port=4
  wires:
  cfblk10/1 -> cfblk15/1, emi_1292/1
  cfblk12/1 -> cyemi_413/1, cyemi_418/1
  cfblk11/1 -> cfblk13/1
  cfblk6/1 -> cyemi_407/1, cyemi_410/1
  cyemi_407/1 -> cfblk10/1
  cfblk5/1 -> cyemi_408/1, emi_1605/1
  cyemi_409/1 -> cfblk17/1
  cfblk9/1 -> cyemi_409/1, emi_62/1
  cyemi_410/1 -> cfblk3/1
  cyemi_411/1 -> cfblk4/1
  cyemi_412/1 -> cfblk5/1
  cfblk4/1 -> cyemi_412/1
  cyemi_413/1 -> cfblk6/1
  cyemi_414/1 -> cfblk6/2
  cfblk1/1 -> cyemi_414/1
  cfblk17/1 -> cyemi_415/1
  cfblk3/1 -> cyemi_416/1
  cyemi_417/1 -> cfblk9/1
  cyemi_418/1 -> cfblk9/2
  cyemi_415/1 -> cfblk7/1(emi_57)
  cfblk7/1(emi_58) -> cyemi_417/1, cfblk2/1
  emi_61/1 -> cfblk7/Action
  emi_61/2 -> emi_59/Action
  emi_62/1 -> emi_61/1
  cyemi_408/1 -> cfblk16/1(emi_1287)
  cfblk16/1(emi_1288) -> cyemi_411/1
  emi_1291/1 -> cfblk16/Action
  emi_1291/2 -> emi_1289/Action
  emi_1292/1 -> emi_1291/1
  cyemi_416/1 -> cfblk8/1(emi_1600)
  cfblk8/1(emi_1601) -> cfblk14/1
  emi_1604/1 -> cfblk8/Action
  emi_1604/2 -> emi_1602/Action
  emi_1605/1 -> emi_1604/1

== system sampleModel7293_pp_1_1/cfblk180 ==
  cfblk1 : Inport
  cfblk14 : Inport  Port=2
  cfblk15 : Inport  Port=3
  cfblk16 : Inport  Port=4
  Action Port : ActionPort  ActionType=then
  cfblk10 : simulink/Discrete/Difference  ICPrevInput=0.0  OutMin=[]  OutMax=[]  OutDataTypeStr=double  OutputDataTypeScalingMode=double  OutDataType=fixdt(1, 16)  OutScaling=2^-10  DoSatur=off
  cfblk11 : DiscreteIntegrator  SampleTime=-1  OutDataTypeStr=double  ICPrevOutput=DiscIntNeverNeededParam  ICPrevScaledInput=DiscIntNeverNeededParam
  cfblk12 : DiscreteFilter
  cfblk13 : If  SampleTime=1
  cfblk17 : Subsystem  TreatAsAtomicUnit=on
  cfblk18 : Subsystem  TreatAsAtomicUnit=on
  cfblk19 : Delay
  cfblk3 : simulink/Continuous/PID Controller  Controller=PID  TimeDomain=Discrete-time  SampleTime=-1  IntegratorMethod=Forward Euler  FilterMethod=Forward Euler  Form=Parallel  UseFilter=on  ControllerParametersSource=internal  P=1  I=1  D=0  N=100  InitialConditionSource=internal  InitialConditionForIntegrator=0  InitialConditionForFilter=0  ExternalReset=none  LimitOutput=off  UpperSaturationLimit=inf  LowerSaturationLimit=-inf  LinearizeAsGain=off  AntiWindupMode=none  Kb=1  TrackingMode=off  Kt=1  PParamMin=[]  PParamMax=[]  IParamMin=[]  IParamMax=[]  DParamMin=[]  DParamMax=[]  NParamMin=[]  NParamMax=[]  KbParamMin=[]  KbParamMax=[]  KtParamMin=[]  KtParamMax=[]  POutMin=[]  POutMax=[]  IOutMin=[]  IOutMax=[]  DOutMin=[]  DOutMax=[]  NOutMin=[]  NOutMax=[]  KbOutMin=[]  KbOutMax=[]  KtOutMin=[]  KtOutMax=[]  IntegratorOutMin=[]  IntegratorOutMax=[]  FilterOutMin=[]  FilterOutMax=[]  SumOutMin=[]  SumOutMax=[]  SumI1OutMin=[]  SumI1OutMax=[]  SumI2OutMin=[]  SumI2OutMax=[]  SumI3OutMin=[]  SumI3OutMax=[]  SumDOutMin=[]  SumDOutMax=[]  SaturationOutMin=[]  SaturationOutMax=[]  IntegratorContinuousStateAttributes=''  IntegratorStateMustResolveToSignalObject=off  IntegratorRTWStateStorageClass=Auto  FilterContinuousStateAttributes=''  FilterStateMustResolveToSignalObject=off  FilterRTWStateStorageClass=Auto  DifferentiatorICPrevScaledInput=0  DifferentiatorOutMin=[]  DifferentiatorOutMax=[]  FilterDiffOutCoefMin=[]  FilterDiffOutCoefMax=[]  SumDenOutMin=[]  SumDenOutMax=[]  SumNumOutMin=[]  SumNumOutMax=[]  ReciprocalOutMin=[]  ReciprocalOutMax=[]  DivideOutMin=[]  DivideOutMax=[]  TunerSelectOption=Transfer Function Based (PID Tuner App)
  cfblk4 : Subsystem  TreatAsAtomicUnit=on
  cfblk5 : UnitDelay  SampleTime=-1
  cfblk6 : simulink/Discrete/Transfer Fcn Lead or Lag  PoleZ=0.95  ZeroZ=0.75  ICPrevOutput=0.0  ICPrevInput=0.0  DoSatur=off
      settings: SourceProductName=Simulink  SourceProductBaseCode=SL
  cfblk7 : DiscreteStateSpace  SampleTime=-1
  cfblk8 : DiscreteZeroPole  Poles=[0 0.5]  Gain=1  SampleTime=-1
  cfblk9 : Subsystem  TreatAsAtomicUnit=on
  cyemi_{424..428,440,455..462} (14 alike) : DataTypeConversion  OutDataTypeStr=double
  emi_2000 : Subsystem  TreatAsAtomicUnit=on
  emi_2002 : If  IfExpression=Inf <= u1
  emi_2003 : DataTypeConversion  OutDataTypeStr=double
  emi_2135 : Subsystem  TreatAsAtomicUnit=on
  emi_2137 : If  IfExpression=Inf <= u1
  emi_2138 : DataTypeConversion  OutDataTypeStr=double
  cfblk2 : Outport
  wires:
  cfblk7/1 -> cfblk2/1
  cfblk13/1 -> cfblk17/Action
  cfblk13/2 -> cfblk18/Action
  cyemi_424/1 -> cfblk10/1
  cfblk5/1 -> cyemi_424/1
  cyemi_425/1 -> cfblk11/1
  cfblk10/1 -> cyemi_425/1
  cyemi_426/1 -> cfblk12/1
  cfblk15/1 -> cyemi_426/1
  cyemi_427/1 -> cfblk13/1
  cfblk16/1 -> cyemi_427/1
  cyemi_428/1 -> cfblk17/1(cfblk1)
  cfblk19/1 -> cyemi_428/1
  cyemi_440/1 -> cfblk18/1(cfblk1)
  cfblk1/1 -> cyemi_440/1
  cyemi_455/1 -> cfblk19/1
  cfblk3/1 -> cyemi_455/1
  cyemi_456/1 -> cfblk3/1
  cfblk18/2(cfblk12) -> cyemi_456/1
  cfblk17/1(cfblk2) -> cyemi_457/1
  cyemi_458/1 -> cfblk5/1
  cfblk18/1(cfblk2) -> cyemi_458/1
  cyemi_459/1 -> cfblk6/1
  cyemi_460/1 -> cfblk7/1
  cfblk12/1 -> cyemi_460/1, emi_2138/1
  cyemi_461/1 -> cfblk8/1
  cfblk8/1 -> cyemi_462/1, emi_2003/1
  cyemi_457/1 -> cfblk4/1(emi_1998)
  cfblk4/1(emi_1999) -> cyemi_461/1
  emi_2002/1 -> cfblk4/Action
  emi_2002/2 -> emi_2000/Action
  emi_2003/1 -> emi_2002/1
  cyemi_462/1 -> cfblk9/1(emi_2133)
  cfblk9/1(emi_2134) -> cyemi_459/1
  emi_2137/1 -> cfblk9/Action
  emi_2137/2 -> emi_2135/Action
  emi_2138/1 -> emi_2137/1
